simulink model "sampleModel2003_1_sub"  (R2023a)
settings: Solver=VariableStepAuto  StartTime=0.0  StopTime=10.0  RelTol=1e-3
libraries: hdlsllib x7, simulink x2
settings Model: Creator=user1  LastModifiedBy=user1

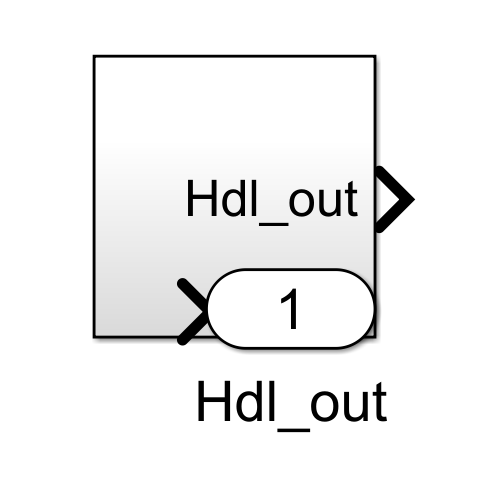
[thumbnail: Simulink's stored preview of the top-level diagram]
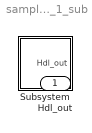
== system sampleModel2003_1_sub ==
  Subsystem : Subsystem
  Hdl_out : Outport  OutDataTypeStr=uint8

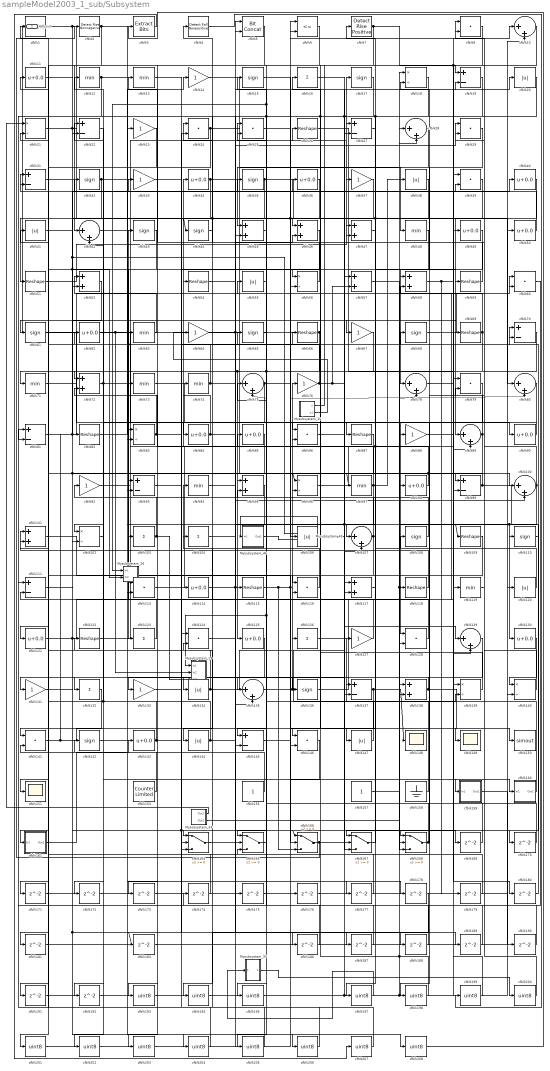
== system sampleModel2003_1_sub/Subsystem ==
  Mysubsystem_15 : Subsystem  TreatAsAtomicUnit=on  RTWFcnName=Mysubsystem_15
      settings: RTWFcnNameOpts=User specified  RTWFileNameOpts=Use function name
  Mysubsystem_19 : Subsystem  TreatAsAtomicUnit=on  RTWFcnName=Mysubsystem_19
      settings: RTWFcnNameOpts=User specified  RTWFileNameOpts=Use function name
  Mysubsystem_26 : Subsystem  TreatAsAtomicUnit=on  RTWFcnName=Mysubsystem_26
      settings: RTWFcnNameOpts=User specified  RTWFileNameOpts=Use function name
  Mysubsystem_33 : Subsystem  TreatAsAtomicUnit=on  RTWFcnName=Mysubsystem_33
      settings: RTWFcnNameOpts=User specified  RTWFileNameOpts=Use function name
  Mysubsystem_35 : Subsystem  TreatAsAtomicUnit=on  RTWFcnName=Mysubsystem_35
      settings: RTWFcnNameOpts=User specified  RTWFileNameOpts=Use function name
  Mysubsystem_45 : Subsystem  TreatAsAtomicUnit=on  RTWFcnName=Mysubsystem_45
      settings: RTWFcnNameOpts=User specified  RTWFileNameOpts=Use function name
  Mysubsystem_46 : Subsystem  TreatAsAtomicUnit=on  RTWFcnName=Mysubsystem_46
      settings: RTWFcnNameOpts=User specified  RTWFileNameOpts=Use function name
  cfblk1 : hdlsllib/Logic and Bit Operations/Compare To Constant  relop=<=  const=3.0  OutDataTypeStr=uint8
  cfblk{10,28,42,75,78,80,89,100,107,129,135} (11 alike) : Sum  Inputs=|++  OutDataTypeStr=uint8
  cfblk{45..47,52,57..58,72,95,101,117,138} (11 alike) : Sum  OutDataTypeStr=uint8
  cfblk{18,21,56,83,96,102,139..140} (8 alike) : Product  Inputs=*/  OutDataTypeStr=uint8  RndMeth=Zero  SaturateOnIntegerOverflow=on
  cfblk{16,103..104,123,126,132} (6 alike) : Sum  Inputs=+  OutDataTypeStr=uint8
  cfblk{20,38,41,55,106,120,134,144,147} (9 alike) : Abs  OutDataTypeStr=uint8  SaturateOnIntegerOverflow=off
  cfblk{15,17,32,35,43..44,61,65,68,108,110,136,142} (13 alike) : Signum
  cfblk{26,51,54,59,66,69,82,87,109,115,118,122} (12 alike) : Reshape
  cfblk{11,34,36,40,49..50,62,84..85,90,98,114,121,125,130,143} (16 alike) : Bias  Bias=0.0  SaturateOnIntegerOverflow=off
  cfblk{19,22,27,31,70,81,93,99,111,137,145} (11 alike) : Sum  Inputs=+-  OutDataTypeStr=uint8
  cfblk{9,24..25,29,39,60,79,86,113,116,124,128,141,146} (14 alike) : DotProduct  OutDataTypeStr=uint8
  cfblk{12..13,48,63,71,73..74,94,97,119} (10 alike) : MinMax  OutDataTypeStr=uint8
  cfblk{14,23,33,37,64,67,76,88,92,127,131,133} (12 alike) : Gain  OutDataTypeStr=uint8
  cfblk148 : Scope
  cfblk149 : Scope
  cfblk150 : ToWorkspace  VariableName=simout  SaveFormat=Timeseries  SampleTime=-1
  cfblk151 : Scope
  cfblk153 : hdlsllib/Sources/Counter Limited  uplimit=7  tsamp=-1
  cfblk155 : Constant  OutDataTypeStr=uint8  SampleTime=-1
  cfblk157 : Constant  OutDataTypeStr=uint8  SampleTime=-1
  cfblk158 : Ground
  cfblk159 : Subsystem
      settings: LibrarySourceBlock=|
      | hdlsllib/Ports &
      | Subsystems/Subsystem
  cfblk160 : Subsystem
      settings: LibrarySourceBlock=|
      | hdlsllib/Ports &
      | Subsystems/Subsystem
  cfblk161 : Subsystem
      settings: LibrarySourceBlock=|
      | hdlsllib/Ports &
      | Subsystems/Subsystem
  cfblk{164..168} (5 alike) : Switch  OutDataTypeStr=uint8  SaturateOnIntegerOverflow=off  InputSameDT=off
  cfblk{169..181,183,186..192} (21 alike) : Delay  SampleTime=1
  cfblk{193..195,197..208} (15 alike) : DataTypeConversion  OutDataTypeStr=uint8  SaturateOnIntegerOverflow=off  RndMeth=Floor
  cfblk2 : hdlsllib/Logic and Bit Operations/Detect Rise Nonnegative  vinit=0  OutDataTypeStr=uint8
  cfblk3 : simulink/Logic and Bit Operations/Extract Bits  bitsToExtract=Upper half  numBits=8  bitIdxRange=[0 7]  outScalingMode=Preserve fixed-point scaling
      settings: LibrarySourceBlock=|
      | hdlsllib/Logic and Bit
      | Operations/Extract Bits
  cfblk4 : hdlsllib/Logic and Bit Operations/Detect Fall Nonpositive  vinit=0  OutDataTypeStr=uint8
  cfblk5 : hdlsllib/Logic and Bit Operations/Bit Concat  numInputs=2
  cfblk6 : RelationalOperator  Operator=<=  OutDataTypeStr=boolean  InputSameDT=off
  cfblk7 : hdlsllib/Logic and Bit Operations/Detect Rise Positive  vinit=0  OutDataTypeStr=uint8
  Hdl_out : Outport  OutDataTypeStr=uint8
  wires:
  cfblk2/1 -> cfblk137/2, cfblk42/1
  cfblk97/1 -> cfblk113/2, cfblk38/1, cfblk34/1
  cfblk121/1 -> cfblk168/3, cfblk60/1
  cfblk122/1 -> cfblk26/1
  cfblk1/1 -> cfblk45/2, cfblk89/1
  cfblk17/1 -> cfblk135/1, cfblk84/1
  cfblk35/1 -> cfblk80/1, cfblk113/1, cfblk144/1
  cfblk126/1 -> cfblk49/1
  cfblk19/1 -> cfblk81/2, cfblk107/1
  cfblk128/1 -> cfblk43/1
  cfblk161/1(Out1) -> cfblk143/1
  cfblk44/1 -> cfblk24/1
  cfblk38/1 -> cfblk134/1
  cfblk51/1 -> cfblk17/1
  cfblk135/1 -> cfblk76/1, cfblk107/2, cfblk139/2
  cfblk85/1 -> cfblk125/1
  cfblk26/1 -> cfblk119/1
  cfblk120/1 -> cfblk92/1
  cfblk107/1 -> cfblk172/1, cfblk25/2
  cfblk66/1 -> Hdl_out/1, cfblk93/2, cfblk95/1
  cfblk42/1 -> cfblk164/1
  cfblk18/1 -> cfblk27/2, cfblk145/2, cfblk116/1
  cfblk25/1 -> cfblk106/1
  cfblk103/1 -> cfblk12/1, Mysubsystem_19/3(In3)
  cfblk46/1 -> cfblk123/1
  cfblk106/1 -> cfblk129/1
  cfblk56/1 -> cfblk13/1
  cfblk59/1 -> cfblk4/1
  cfblk99/1 -> cfblk93/1, cfblk167/1
  cfblk166/1 -> cfblk70/1, cfblk2/1
  cfblk52/1 -> cfblk121/1
  cfblk80/1 -> cfblk128/1
  cfblk88/1 -> cfblk160/1(In1)
  cfblk48/1 -> cfblk78/1
  cfblk134/1 -> cfblk126/1, cfblk21/2
  cfblk40/1 -> cfblk161/1(In1), cfblk87/1
  cfblk63/1 -> cfblk52/1
  cfblk43/1 -> cfblk131/1
  cfblk50/1 -> cfblk11/1
  cfblk86/1 -> cfblk98/1
  cfblk113/1 -> cfblk40/1
  cfblk117/1 -> cfblk7/1
  cfblk96/1 -> cfblk28/1
  cfblk136/1 -> cfblk88/1
  cfblk137/1 -> cfblk146/2, cfblk148/1
  cfblk100/1 -> cfblk47/2, cfblk128/2, cfblk130/1
  cfblk34/1 -> cfblk203/1, cfblk138/1
  cfblk72/1 -> cfblk22/1, cfblk54/1
  cfblk24/1 -> cfblk83/2, cfblk117/2
  cfblk98/1 -> cfblk96/1, cfblk47/1, cfblk73/1
  cfblk64/1 -> cfblk20/1, cfblk100/1
  cfblk133/1 -> cfblk39/2
  cfblk39/1 -> cfblk56/2, cfblk44/1
  cfblk102/1 -> cfblk132/1
  cfblk7/1 -> cfblk19/1, cfblk56/1
  cfblk79/1 -> cfblk198/1
  cfblk155/1 -> cfblk101/1
  cfblk70/1 -> cfblk71/1
  cfblk81/1 -> cfblk36/1, cfblk55/1
  cfblk90/1 -> cfblk83/1
  cfblk61/1 -> cfblk86/1
  cfblk11/1 -> cfblk164/3, cfblk97/1, Mysubsystem_26/2(In2)
  cfblk157/1 -> cfblk28/2
  cfblk62/1 -> cfblk115/1, Mysubsystem_19/2(In2)
  cfblk143/1 -> cfblk68/1, cfblk42/2
  cfblk89/1 -> cfblk167/3, cfblk33/1
  cfblk95/1 -> cfblk133/1
  cfblk139/1 -> cfblk16/1
  cfblk130/1 -> cfblk140/1
  cfblk141/1 -> cfblk82/1, cfblk149/1
  cfblk94/1 -> cfblk100/2
  cfblk68/1 -> cfblk60/2
  cfblk118/1 -> cfblk101/2
  cfblk33/1 -> cfblk59/1
  cfblk140/1 -> cfblk9/1
  cfblk32/1 -> cfblk177/1, cfblk102/2
  cfblk76/1 -> cfblk31/2, cfblk63/1, cfblk57/2, cfblk19/2
  cfblk92/1 -> cfblk85/1
  cfblk37/1 -> cfblk51/1
  cfblk16/1 -> cfblk109/1, cfblk168/1
  cfblk147/1 -> cfblk127/1
  cfblk153/1 -> cfblk142/1
  cfblk31/1 -> cfblk114/1
  cfblk167/1 -> cfblk37/1
  cfblk21/1 -> cfblk46/1, cfblk206/1, cfblk183/1
  cfblk78/1 -> cfblk10/1
  cfblk20/1 -> cfblk146/1
  cfblk75/1 -> cfblk192/1, cfblk99/1
  cfblk84/1 -> cfblk74/1, cfblk66/1
  cfblk69/1 -> cfblk58/2, cfblk205/1, cfblk103/1
  cfblk82/1 -> cfblk14/1
  cfblk168/1 -> cfblk108/1, cfblk65/1
  cfblk71/1 -> cfblk50/1
  cfblk47/1 -> cfblk147/1
  cfblk116/1 -> cfblk94/1
  cfblk9/1 -> cfblk99/2, cfblk61/1
  cfblk125/1 -> cfblk141/1
  cfblk45/1 -> cfblk165/1
  cfblk123/1 -> cfblk41/1
  cfblk115/1 -> cfblk166/3, cfblk80/2, cfblk159/1(In1)
  cfblk13/1 -> cfblk67/1
  cfblk93/1 -> cfblk164/2
  cfblk10/1 -> cfblk75/2, Mysubsystem_26/1(In1)
  cfblk12/1 -> cfblk22/2, cfblk23/1
  cfblk114/1 -> cfblk188/1, cfblk29/2
  cfblk145/1 -> cfblk9/2
  cfblk87/1 -> cfblk151/1
  cfblk73/1 -> cfblk129/2
  cfblk144/1 -> cfblk27/1, cfblk31/1, cfblk122/1
  cfblk28/1 -> cfblk45/1
  cfblk119/1 -> cfblk29/1
  cfblk15/1 -> cfblk90/1
  cfblk108/1 -> cfblk35/1
  cfblk14/1 -> cfblk48/1
  cfblk127/1 -> cfblk104/1
  cfblk22/1 -> cfblk102/1
  cfblk104/1 -> cfblk46/2
  cfblk67/1 -> cfblk72/1
  cfblk55/1 -> cfblk25/1
  cfblk138/1 -> cfblk136/1, cfblk150/1
  cfblk54/1 -> cfblk110/1
  cfblk83/1 -> cfblk72/2, cfblk186/1, cfblk166/1
  cfblk41/1 -> cfblk69/1, Mysubsystem_45/1(In1)
  cfblk158/1 -> cfblk137/1
  cfblk160/1(Out1) -> cfblk32/1
  cfblk74/1 -> cfblk135/2, cfblk62/1
  cfblk36/1 -> cfblk52/2
  cfblk29/1 -> cfblk58/1
  cfblk6/1 -> cfblk193/1
  cfblk58/1 -> cfblk180/1, cfblk179/1
  cfblk65/1 -> cfblk15/1
  cfblk101/1 -> cfblk166/2
  cfblk57/1 -> cfblk169/1
  cfblk169/1 -> cfblk18/2
  cfblk110/1 -> cfblk170/1
  cfblk170/1 -> cfblk95/2
  cfblk132/1 -> cfblk171/1
  cfblk171/1 -> cfblk10/2
  cfblk172/1 -> cfblk24/2
  cfblk129/1 -> cfblk173/1
  cfblk173/1 -> cfblk89/2
  cfblk60/1 -> cfblk174/1
  cfblk174/1 -> cfblk1/1
  cfblk164/1 -> cfblk175/1
  cfblk175/1 -> cfblk39/1
  cfblk176/1 -> cfblk96/2
  cfblk177/1 -> cfblk75/1
  cfblk124/1 -> cfblk178/1
  cfblk179/1 -> cfblk141/2
  cfblk180/1 -> cfblk70/2
  cfblk23/1 -> cfblk181/1
  cfblk181/1 -> cfblk117/1
  cfblk183/1 -> cfblk140/2
  cfblk186/1 -> cfblk165/3
  cfblk27/1 -> cfblk187/1
  cfblk187/1 -> cfblk81/1
  cfblk188/1 -> cfblk167/2
  cfblk131/1 -> cfblk189/1
  cfblk189/1 -> cfblk168/2
  cfblk159/1(Out1) -> cfblk190/1
  cfblk190/1 -> cfblk116/2
  cfblk109/1 -> cfblk191/1
  cfblk191/1 -> cfblk139/1
  cfblk192/1 -> cfblk165/2
  cfblk193/1 -> cfblk57/1, cfblk120/1, cfblk78/2, cfblk118/1
  cfblk178/1 -> cfblk194/1
  cfblk194/1 -> cfblk6/1
  cfblk165/1 -> cfblk195/1
  cfblk195/1 -> cfblk6/2
  cfblk49/1 -> cfblk197/1
  cfblk198/1 -> cfblk18/1, cfblk86/2
  cfblk4/1 -> cfblk199/1
  cfblk199/1 -> cfblk79/1
  cfblk200/1 -> cfblk79/2
  cfblk5/1 -> cfblk201/1
  cfblk201/1 -> cfblk176/1
  cfblk146/1 -> cfblk202/1
  cfblk202/1 -> cfblk5/1
  cfblk203/1 -> cfblk5/2
  cfblk111/1 -> cfblk204/1
  cfblk204/1 -> cfblk124/1
  cfblk205/1 -> cfblk111/1
  cfblk206/1 -> cfblk111/2
  cfblk3/1 -> cfblk207/1
  cfblk207/1 -> cfblk124/2
  cfblk142/1 -> cfblk208/1
  cfblk208/1 -> cfblk3/1
  Mysubsystem_15/1(y) -> cfblk145/1, Mysubsystem_19/1(In1)
  Mysubsystem_15/2(y1) -> cfblk64/1
  Mysubsystem_33/1(Out1) -> cfblk21/1
  Mysubsystem_33/2(Out2) -> cfblk138/2
  cfblk197/1 -> Mysubsystem_35/1(In1)
  Mysubsystem_35/1(Out1) -> cfblk200/1
  Mysubsystem_45/1(Out1) -> Mysubsystem_46/1(In1)
  Mysubsystem_46/1(Out1) -> Mysubsystem_45/2(In2)

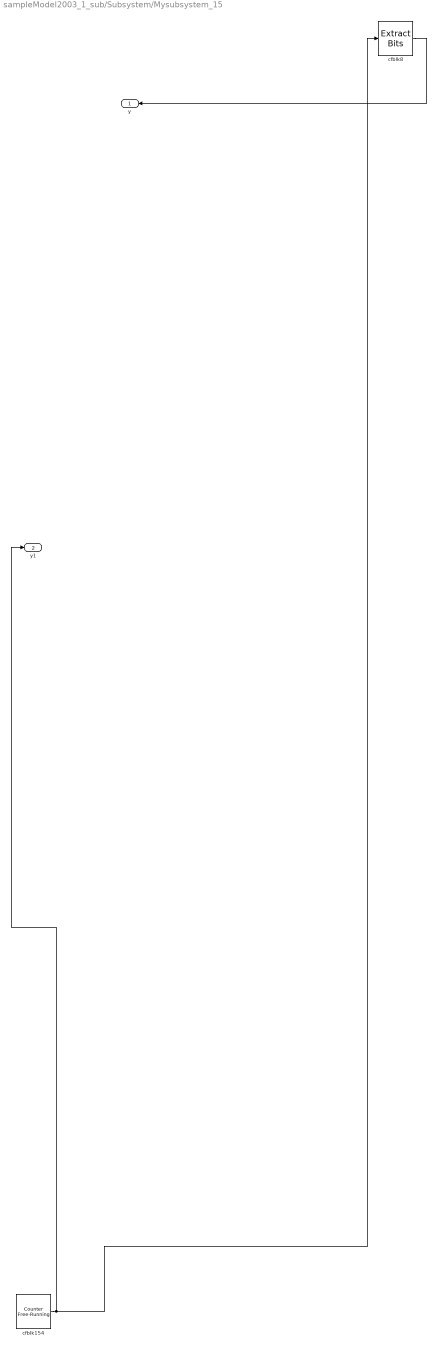
== system sampleModel2003_1_sub/Subsystem/Mysubsystem_15 ==
  cfblk154 : hdlsllib/Sources/Counter Free-Running  NumBits=16  tsamp=-1
  cfblk8 : simulink/Logic and Bit Operations/Extract Bits  bitsToExtract=Upper half  numBits=8  bitIdxRange=[0 7]  outScalingMode=Preserve fixed-point scaling
      settings: LibrarySourceBlock=|
      | hdlsllib/Logic and Bit
      | Operations/Extract Bits
  y : Outport
  y1 : Outport  Port=2
  wires:
  cfblk154/1 -> cfblk8/1, y1/1
  cfblk8/1 -> y/1

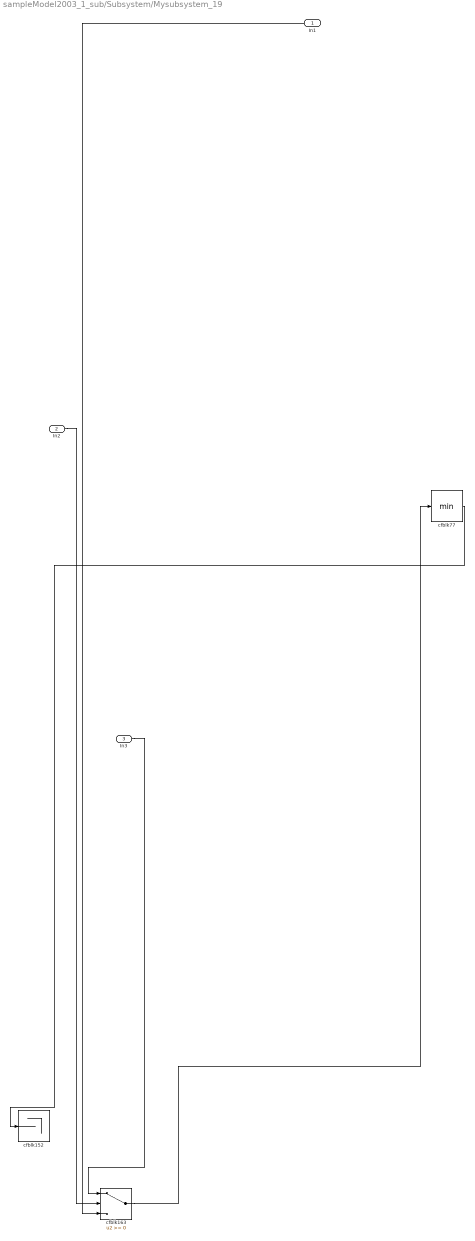
== system sampleModel2003_1_sub/Subsystem/Mysubsystem_19 ==
  In1 : Inport
  In2 : Inport  Port=2
  In3 : Inport  Port=3
  cfblk152 : Terminator
  cfblk163 : Switch  SaturateOnIntegerOverflow=off  InputSameDT=off
  cfblk77 : MinMax
  wires:
  In2/1 -> cfblk163/2
  In3/1 -> cfblk163/1
  In1/1 -> cfblk163/3
  cfblk163/1 -> cfblk77/1
  cfblk77/1 -> cfblk152/1

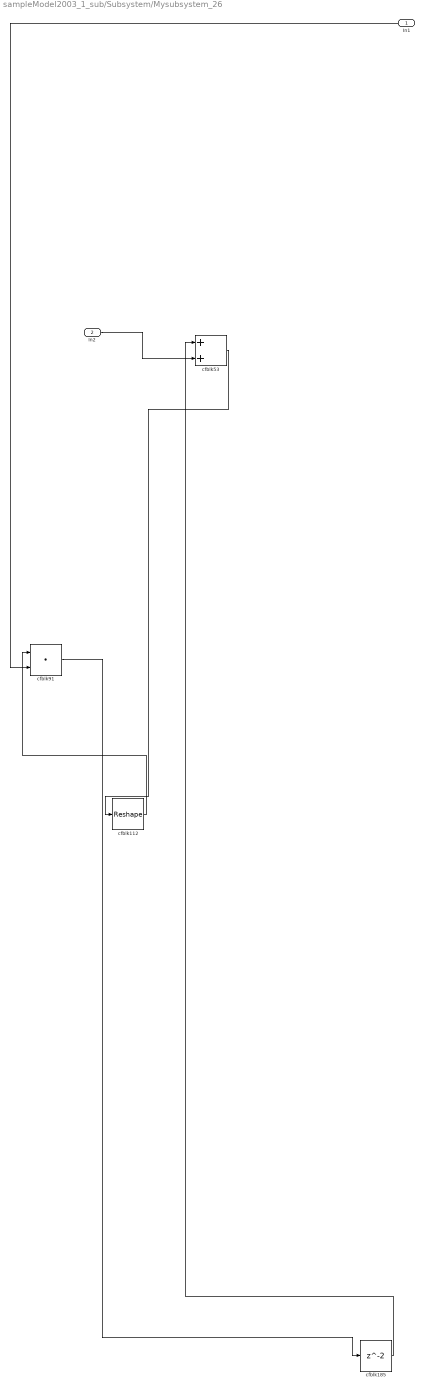
== system sampleModel2003_1_sub/Subsystem/Mysubsystem_26 ==
  In1 : Inport
  In2 : Inport  Port=2
  cfblk112 : Reshape
  cfblk185 : Delay  SampleTime=1
  cfblk53 : Sum
  cfblk91 : DotProduct  OutDataTypeStr=Inherit: Inherit via internal rule
  wires:
  In2/1 -> cfblk53/2
  cfblk91/1 -> cfblk185/1
  cfblk53/1 -> cfblk112/1
  cfblk185/1 -> cfblk53/1
  In1/1 -> cfblk91/2
  cfblk112/1 -> cfblk91/1

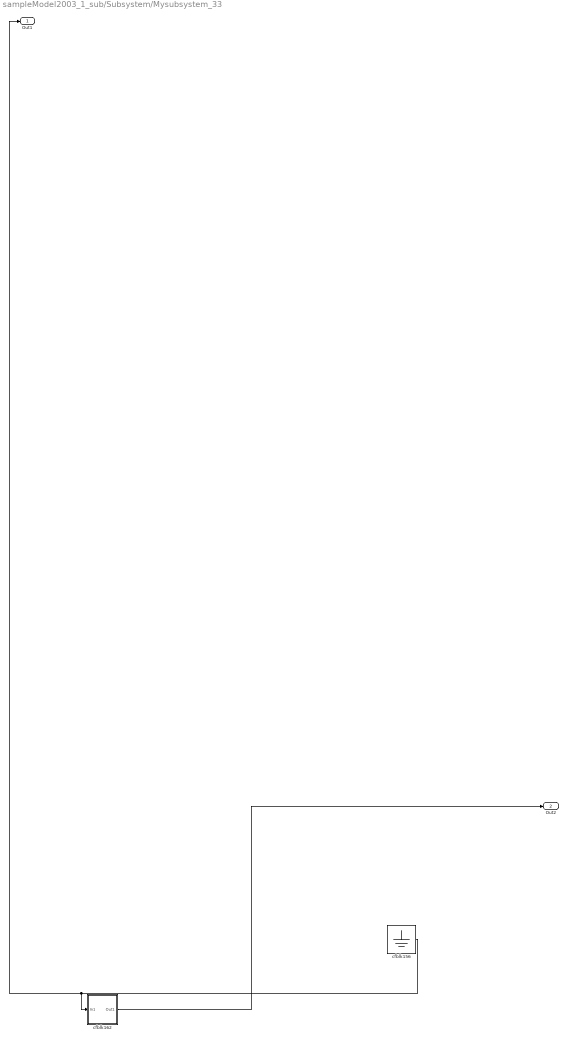
== system sampleModel2003_1_sub/Subsystem/Mysubsystem_33 ==
  cfblk156 : Ground
  cfblk162 : Subsystem
      settings: LibrarySourceBlock=|
      | hdlsllib/Ports &
      | Subsystems/Subsystem
  Out1 : Outport
  Out2 : Outport  Port=2
  wires:
  cfblk156/1 -> cfblk162/1(In1), Out1/1
  cfblk162/1(Out1) -> Out2/1

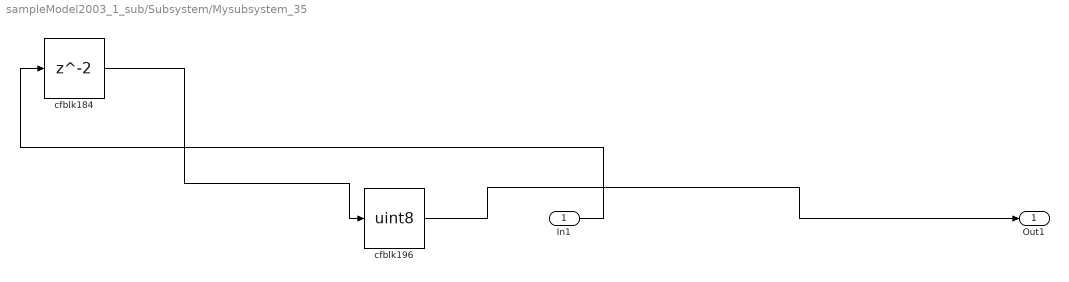
== system sampleModel2003_1_sub/Subsystem/Mysubsystem_35 ==
  In1 : Inport
  cfblk184 : Delay  SampleTime=1
  cfblk196 : DataTypeConversion  OutDataTypeStr=uint8  SaturateOnIntegerOverflow=off  RndMeth=Floor
  Out1 : Outport
  wires:
  cfblk196/1 -> Out1/1
  In1/1 -> cfblk184/1
  cfblk184/1 -> cfblk196/1

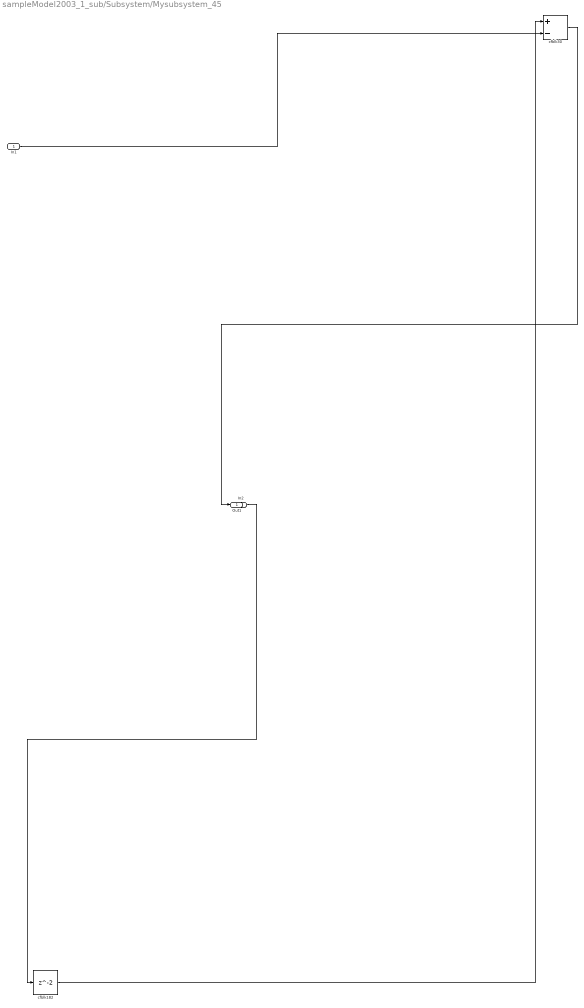
== system sampleModel2003_1_sub/Subsystem/Mysubsystem_45 ==
  In1 : Inport
  In2 : Inport  Port=2
  cfblk182 : Delay  SampleTime=1
  cfblk30 : Sum  Inputs=+-
  Out1 : Outport
  wires:
  In2/1 -> cfblk182/1
  cfblk30/1 -> Out1/1
  In1/1 -> cfblk30/2
  cfblk182/1 -> cfblk30/1

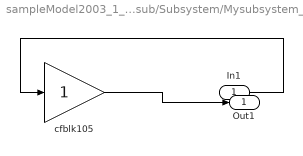
== system sampleModel2003_1_sub/Subsystem/Mysubsystem_46 ==
  In1 : Inport
  cfblk105 : Gain
  Out1 : Outport
  wires:
  cfblk105/1 -> Out1/1
  In1/1 -> cfblk105/1

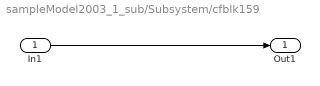
== system sampleModel2003_1_sub/Subsystem/cfblk159 ==
  In1 : Inport
  Out1 : Outport
  wires:
  In1/1 -> Out1/1

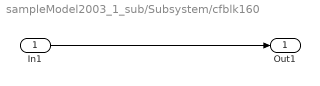
== system sampleModel2003_1_sub/Subsystem/cfblk160 ==
  In1 : Inport
  Out1 : Outport
  wires:
  In1/1 -> Out1/1

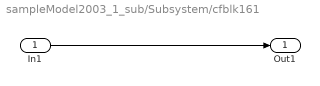
== system sampleModel2003_1_sub/Subsystem/cfblk161 ==
  In1 : Inport
  Out1 : Outport
  wires:
  In1/1 -> Out1/1

== system sampleModel2003_1_sub/Subsystem/Mysubsystem_33/cfblk162 ==
  In1 : Inport
  Out1 : Outport
  wires:
  In1/1 -> Out1/1
